simulink model "MazeGame_full"  (R2021b)
settings: Solver=FixedStepDiscrete  StartTime=0.0  StopTime=inf  FixedStep=0.001  RelTol=1e-3  EnableMultiTasking=on
PreLoadFcn:
  | initParameter;
values from neighbouring files (symbols this model uses):
  Angular2Linear = (0.054/(2*pi))    (= 0.00859436692696)    [initParameter_pendulum.m]
  cmdEl72x1_ENABLE_OPERATION = bin2dec('0000 0000 0000 1111')    [initStateMachine.m]
  cmdEl72x1_FAULT_RESET = bin2dec('0000 0000 1000 0000')    [initStateMachine.m]
  cmdEl72x1_STOP = bin2dec('0000 0000 0000 0000')    [initStateMachine.m]
  cmdEl72x1_SWITCH_ON = bin2dec('0000 0000 0000 0111')    [initStateMachine.m]
  cmdEl72x1_VOLTAGE_AND_RELEASE = bin2dec('0000 0000 0000 0110')    [initStateMachine.m]
  Counts2Voltage = (SupplyVoltage_Bottom/(32767*0.5))    (= 0.00030518509476)    [initParameter_pendulum.m]
  Counts2Voltage_top = (SupplyVoltage_Top/(32767*0.5))    (= 0.00030518509476)    [initParameter_pendulum.m]
  gearRatio_Motor1 = 1/1    (= 1)    [initParameter.m]    (also in initParameter_pendulum.m)
  increments2rad_AM8113_0F21 = 2*pi/2^20    (= 5.99211245268e-06)    [initParameter_pendulum.m]
  increments2radPerS_AM8113_0F21 = 2*pi/268435    (= 2.340672903e-05)    [initParameter_pendulum.m]
  output2Torque_AM8113_0F21 = ((1/1000)*(ratedCurrent_AM8113_0F21/sqrt(2)))*torqueConstant_AM8113_0F21    [initParameter_pendulum.m]
  PointZero_Bottom = 2476    [initParameter_pendulum.m]
  PointZero_Top = (19584 - 6*pi)    (= 19565.1504441)    [initParameter_pendulum.m]
  Safe_Distance = 0.2    [initParameter_pendulum.m]
  SupplyVoltage_Bottom = 5    [initParameter_pendulum.m]
  SupplyVoltage_Top = 5    [initParameter_pendulum.m]
  Velocity_Limit = 80*pi    (= 251.327412287)    [initParameter_pendulum.m]
  vmax_AM8113_0F21 = 90*pi    (= 282.743338823)    [initParameter_pendulum.m]
  vmin_AM8113_0F21 = -90*pi    (= -282.743338823)    [initParameter_pendulum.m]
  Voltage2Angle = SupplyVoltage_Bottom/(2*pi)    (= 0.795774715459)    [initParameter_pendulum.m]
  Voltage2Angle_top = 4.3/(2*pi)    (= 0.684366255295)    [initParameter_pendulum.m]
  Voltage2Counts = (32766/10)    (= 3276.6)    [initParameter_pendulum.m]
  x_11 = PointZero_Bottom - 1.5*pi    (= 2471.28761102)    [initParameter_pendulum.m]
  x_12 = PointZero_Bottom - (20*2*pi) + (4*2*pi)    (= 2375.46903509)    [initParameter_pendulum.m]
  x_21 = PointZero_Top + (3*2*pi)    (= 19584)    [initParameter_pendulum.m]
  x_22 = PointZero_Top + (20*2*pi)    (= 19690.8141502)    [initParameter_pendulum.m]
libraries: simulink x13, cstblocks x2
settings Model: SimulationMode=external  Creator=rauterg  LastModifiedBy=BIROMED-Lab
settings SolverCC: AlgebraicLoopSolver=TrustRegion
settings DataIOCC: LimitDataPoints=on  SaveFormat=Array  SignalLoggingSaveFormat=ModelDataLogs  ReturnWorkspaceOutputs=off
settings OptimizationCC: BlockReduction=off  ConditionallyExecuteInputs=off  UseDivisionForNetSlopeComputation=UseDivisionForReciprocalsOfIntegersOnly  OptimizeBlockIOStorage=off  BufferReuse=off  GlobalBufferReuse=off  ExpressionFolding=off  ExpressionDepthLimit=2147483647  LocalBlockOutputs=off  EfficientFloat2IntCast=on  OptimizeDataStoreBuffers=off  BusAssignmentInplaceUpdate=off
settings DebuggingCC: ConsistencyChecking=warning  SignalInfNanChecking=warning  SignalRangeChecking=error  ReadBeforeWriteMsg=EnableAllAsError  WriteAfterWriteMsg=EnableAllAsError  WriteAfterReadMsg=EnableAllAsError  AlgebraicLoopMsg=error  UnderspecifiedInitializationDetection=Classic  MergeDetectMultiDrivingBlocksExec=none  CheckExecutionContextPreStartOutputMsg=on  BlockPriorityViolationMsg=error  MinStepSizeMsg=error  TimeAdjustmentMsg=warning  SolverPrmCheckMsg=error  SigSpecEnsureSampleTimeMsg=error  CheckMatrixSingularityMsg=error  IntegerOverflowMsg=error  ParameterUnderflowMsg=error  ParameterPrecisionLossMsg=error  ParameterTunabilityLossMsg=error  UnderSpecifiedDataTypeMsg=error  UnnecessaryDatatypeConvMsg=warning  VectorMatrixConversionMsg=error  FcnCallInpInsideContextMsg=warning  SignalLabelMismatchMsg=error  UnconnectedInputMsg=error  UnconnectedOutputMsg=error  UnconnectedLineMsg=error  SFcnCompatibilityMsg=warning  UniqueDataStoreMsg=error  BusObjectLabelMismatch=error  RootOutportRequireBusObject=error  AssertControl=DisableAll  ModelReferenceIOMsg=error  ModelReferenceIOMismatchMessage=error  UnknownTsInhSupMsg=error  ModelReferenceDataLoggingMessage=error  StateNameClashWarn=warning  StrictBusMsg=ErrorOnBusTreatedAsVector  SFUnexpectedBacktrackingDiag=warning  SFNoUnconditionalDefaultTransitionDiag=warning  SFExecutionAtInitializationDiag=none  SFMachineParentedDataDiag=warning  IntegerSaturationMsg=error  ArithmeticOperatorsInVariantConditions=warning
settings HardwareCC: ProdBitPerPointer=32  ProdBitPerSizeT=32  ProdBitPerPtrDiffT=32  ProdLargestAtomicFloat=None  ProdWordSize=32  ProdLongLongMode=on  ProdHWDeviceType=Generic->32-bit x86 compatible
settings ModelReferenceCC: PropagateSignalLabelsOutOfModel=off
settings SFSimCC: SimUseLocalCustomCode=off  CustomCodeUndefinedFunction=UseInterfaceOnly  SimTargetLang=C++
settings RTWCC: Description=TwinCAT GRT Target  SystemTargetFile=TwinCatGrt.tlc  GenCodeOnly=on  TemplateMakefile=tcgrt_msbuild.tmf  GenerateReport=on  RTWUseLocalCustomCode=off  TargetLang=C++
settings CodeAppCC: ForceParamTrailComments=on  MangleLength=4  StateflowObjectComments=on  MATLABSourceComments=on
settings STFCustomTargetCC: TargetLangStandard=C++11 (ISO)  CombineOutputUpdateFcns=on  CodeInterfacePackaging=Reusable function  CPPClassGenCompliant=on  GRTInterface=off  GenerateAllocFcn=on  SystemTargetFile=TwinCatGrt.tlc
settings GRTTargetCC: TargetLangStandard=C++11 (ISO)  ParMdlRefBuildCompliant=off  CompOptLevelCompliant=off  ConcurrentExecutionCompliant=off  MatFileLogging=off  CodeInterfacePackaging=Reusable function  GenerateAllocFcn=on  UseToolchainInfoCompliant=off  ExtModeMexFile=TcExtModeClient
settings ConfigComp: CovMetricSettings=dw  CovSaveCumulativeToWorkspaceVar=on  CovSaveSingleToWorkspaceVar=on  CovExternalEMLEnable=off

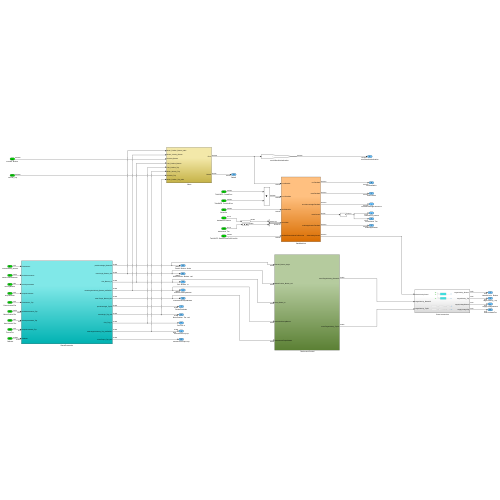
[thumbnail: Simulink's stored preview of the top-level diagram]
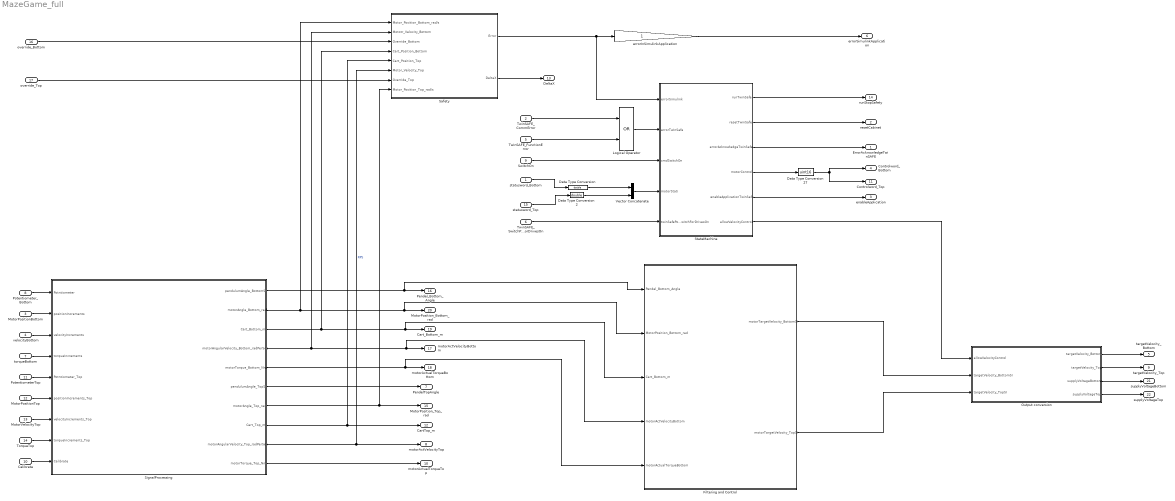
== system MazeGame_full ==
  statusword_Bottom : Inport  OutDataTypeStr=uint16
  TwinSAFE_CommError : Inport  Port=2  OutDataTypeStr=boolean
  MotorPositionBottom : Inport  Port=3  OutDataTypeStr=uint32
  velocityBottom : Inport  Port=4  OutDataTypeStr=int32
  TwinSAFE_FunctionError : Inport  Port=5  OutDataTypeStr=boolean
  TwinSAFE_SwitchPowerForDrivesOn : Inport  Port=6  OutDataTypeStr=boolean
  torqueBottom : Inport  Port=7  OutDataTypeStr=int16
  Potentiometer_Bottom : Inport  Port=8  OutDataTypeStr=int16
  SwitchOn : Inport  Port=9  OutDataTypeStr=boolean
  Calibrate : Inport  Port=10  OutDataTypeStr=boolean
  PotentiometerTop : Inport  Port=11  OutDataTypeStr=int16
  MotorPositionTop : Inport  Port=12  OutDataTypeStr=uint32
  MotorVelocityTop : Inport  Port=13  OutDataTypeStr=int32
  TorqueTop : Inport  Port=14  OutDataTypeStr=int16
  statusword_Top : Inport  Port=15  OutDataTypeStr=uint16
  override_Bottom : Inport  Port=16  OutDataTypeStr=boolean
  override_Top : Inport  Port=17  OutDataTypeStr=boolean
  Data Type Conversion : DataTypeConversion  OutDataTypeStr=double
  Data Type Conversion2 : DataTypeConversion  OutDataTypeStr=double
  Data Type Conversion27 : DataTypeConversion  OutDataTypeStr=uint16
  Filtering and Control : Subsystem
  Logical Operator : Logic  Operator=OR  AllPortsSameDT=off  OutDataTypeStr=boolean
  Output conversion : Subsystem
  Safety : Subsystem
  SignalProcessing : Subsystem
  StateMachine : Subsystem
  Vector Concatenate : Concatenate
  errorInSimulinkApplication : Gain  OutDataTypeStr=Inherit: Same as input
  ErrorAcknowledgeTwinSAFE : Outport  OutDataTypeStr=boolean  VectorParamsAs1DForOutWhenUnconnected=off
  resetCabinet : Outport  Port=2  OutDataTypeStr=boolean  VectorParamsAs1DForOutWhenUnconnected=off
  enableApplication : Outport  Port=3  OutDataTypeStr=boolean  VectorParamsAs1DForOutWhenUnconnected=off
  Controlword_Bottom : Outport  Port=4  OutDataTypeStr=uint16  VectorParamsAs1DForOutWhenUnconnected=off
  targetVelocity_Bottom : Outport  Port=5  OutDataTypeStr=int32  PortDimensions=1  VectorParamsAs1DForOutWhenUnconnected=off
  errorSimulinkApplication : Outport  Port=6  OutDataTypeStr=boolean  VectorParamsAs1DForOutWhenUnconnected=off
  PendelTopAngle : Outport  Port=7  OutDataTypeStr=double  VectorParamsAs1DForOutWhenUnconnected=off
  motorActVelocityTop : Outport  Port=8  OutDataTypeStr=double  VectorParamsAs1DForOutWhenUnconnected=off
  targetVelocity_Top : Outport  Port=9  OutDataTypeStr=int32  PortDimensions=1  VectorParamsAs1DForOutWhenUnconnected=off
  motorActualTorqueTop : Outport  Port=10  VectorParamsAs1DForOutWhenUnconnected=off
  Controlword_Top : Outport  Port=11  OutDataTypeStr=uint16  VectorParamsAs1DForOutWhenUnconnected=off
  CartTop_m : Outport  Port=12  VectorParamsAs1DForOutWhenUnconnected=off
  DeltaX : Outport  Port=13  OutDataTypeStr=double  VectorParamsAs1DForOutWhenUnconnected=off
  runStopSafety : Outport  Port=14  OutDataTypeStr=boolean  VectorParamsAs1DForOutWhenUnconnected=off
  MotorPosition_Top_rad : Outport  Port=15  OutDataTypeStr=double  VectorParamsAs1DForOutWhenUnconnected=off
  Pendel_Bottom_Angle : Outport  Port=16  OutDataTypeStr=double  VectorParamsAs1DForOutWhenUnconnected=off
  motorActVelocityBottom : Outport  Port=17  OutDataTypeStr=double  VectorParamsAs1DForOutWhenUnconnected=off
  motorActualTorqueBottom : Outport  Port=18  VectorParamsAs1DForOutWhenUnconnected=off
  Cart_Bottom_m : Outport  Port=19  VectorParamsAs1DForOutWhenUnconnected=off
  MotorPosition_Bottom_rad : Outport  Port=20  OutDataTypeStr=double  VectorParamsAs1DForOutWhenUnconnected=off
  supplyVoltageBottom : Outport  Port=21  OutDataTypeStr=int16  PortDimensions=1  VectorParamsAs1DForOutWhenUnconnected=off
  supplyVoltageTop : Outport  Port=22  OutDataTypeStr=int16  PortDimensions=1  VectorParamsAs1DForOutWhenUnconnected=off
  wires:
  TwinSAFE_CommError/1 -> Logical Operator/1
  TwinSAFE_FunctionError/1 -> Logical Operator/2
  Logical Operator/1 -> StateMachine/2(errorTwinSafe)
  SignalProcessing/4(motorAngularVelocity_Bottom_radPerSec) -> Filtering and Control/4(motorActVelocityBottom), motorActVelocityBottom/1, Safety/2(Mototr_Velocity_Bottom)
  Data Type Conversion27/1 -> Controlword_Bottom/1, Controlword_Top/1
  errorInSimulinkApplication/1 -> errorSimulinkApplication/1
  TwinSAFE_SwitchPowerForDrivesOn/1 -> StateMachine/5(twinSafePowerSwitchForDrivesOn)
  StateMachine/5(enableApplicationTwinSafe) -> enableApplication/1
  StateMachine/2(resetTwinSafe) -> resetCabinet/1
  MotorPositionBottom/1 -> SignalProcessing/2(positionIncrements)
  velocityBottom/1 -> SignalProcessing/3(velocityIncrements)
  torqueBottom/1 -> SignalProcessing/4(torqueIncrements)
  SignalProcessing/5(motorTorque_Bottom_Nm) -> Filtering and Control/5(motorActualTorqueBottom), motorActualTorqueBottom/1
  Potentiometer_Bottom/1 -> SignalProcessing/1(Potntiometer)
  SwitchOn/1 -> StateMachine/3(cmdSwitchOn)
  Calibrate/1 -> SignalProcessing/9(Calibrate)
  SignalProcessing/3(Cart_Bottom_m) -> Filtering and Control/3(Cart_Bottom_m), Cart_Bottom_m/1, Safety/4(Cart_Position_Bottom)
  SignalProcessing/1(pendulumAngle_BottomSI) -> Filtering and Control/1(Pendel_Bottom_Angle), Pendel_Bottom_Angle/1
  PotentiometerTop/1 -> SignalProcessing/5(Potntiometer_Top)
  SignalProcessing/6(pendulumAngle_TopSI) -> PendelTopAngle/1
  SignalProcessing/7(motorAngle_Top_rad) -> MotorPosition_Top_rad/1, Safety/8(Motor_Position_Top_rad/s)
  SignalProcessing/9(motorAngularVelocity_Top_radPerSec) -> motorActVelocityTop/1, Safety/6(Motor_Velocity_Top)  "RPS"
  SignalProcessing/10(motorTorque_Top_Nm) -> motorActualTorqueTop/1
  SignalProcessing/8(Cart_Top_m) -> CartTop_m/1, Safety/5(Cart_Position_Top)
  MotorPositionTop/1 -> SignalProcessing/6(positionIncrements_Top)
  MotorVelocityTop/1 -> SignalProcessing/7(velocityIncrements_Top)
  TorqueTop/1 -> SignalProcessing/8(torqueIncrements_Top)
  Data Type Conversion/1 -> Vector Concatenate/1
  statusword_Bottom/1 -> Data Type Conversion/1
  statusword_Top/1 -> Data Type Conversion2/1
  StateMachine/4(motorControl) -> Data Type Conversion27/1
  StateMachine/3(errorAcknowledgeTwinSafe) -> ErrorAcknowledgeTwinSAFE/1
  Data Type Conversion2/1 -> Vector Concatenate/2
  Safety/1(Error) -> StateMachine/1(errorSimulink), errorInSimulinkApplication/1
  Safety/2(DeltaX) -> DeltaX/1
  Vector Concatenate/1 -> StateMachine/4(motorStati)
  StateMachine/1(runTwinSafe) -> runStopSafety/1
  Output conversion/1("targetVelocity_Bottom ") -> targetVelocity_Bottom/1
  Output conversion/2(targetVelocity_Top) -> targetVelocity_Top/1
  Filtering and Control/1(motorTargetVelocity_BottomSI) -> Output conversion/2(targetVelocity_BottomSI)
  Filtering and Control/2(motorTargetVelocity_TopSI) -> Output conversion/3(targetVelocity_TopSI)
  SignalProcessing/2(motorAngle_Bottom_rad) -> MotorPosition_Bottom_rad/1, Filtering and Control/2(MotorPosition_Bottom_rad), Safety/1(Motor_Position_Bottom_rad/s)
  override_Top/1 -> Safety/7(Override_Top)
  override_Bottom/1 -> Safety/3(Override_Bottom)
  StateMachine/6(allowVelocityControl) -> Output conversion/1(allowVelocityControl)
  Output conversion/4(supplyVoltageTop) -> supplyVoltageTop/1
  Output conversion/3(supplyVoltageBottom) -> supplyVoltageBottom/1

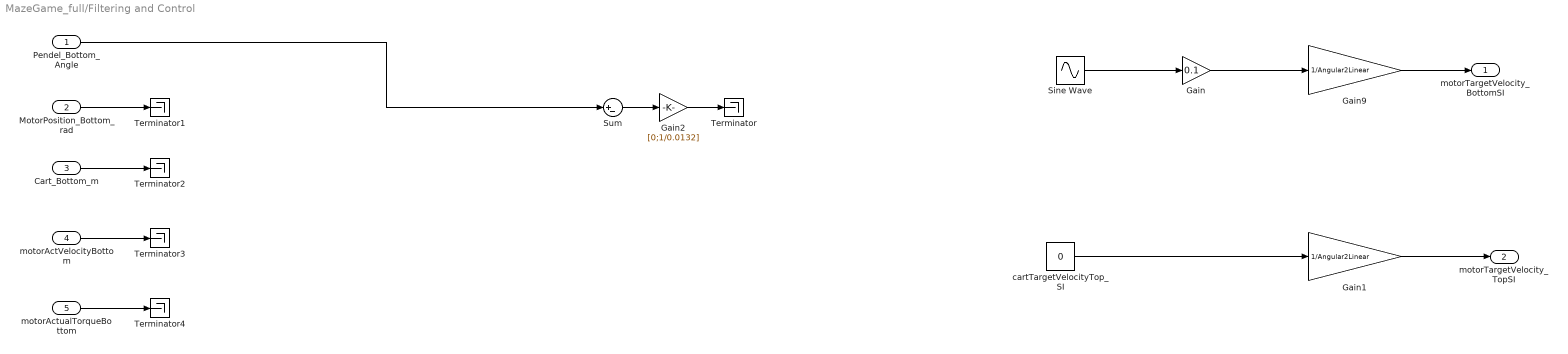
== system MazeGame_full/Filtering and Control ==
  Pendel_Bottom_Angle : Inport  OutDataTypeStr=double
  MotorPosition_Bottom_rad : Inport  Port=2  OutDataTypeStr=double
  Cart_Bottom_m : Inport  Port=3  OutDataTypeStr=double
  motorActVelocityBottom : Inport  Port=4  OutDataTypeStr=double
  motorActualTorqueBottom : Inport  Port=5  OutDataTypeStr=double
  Gain : Gain  Gain=0.1
  Gain1 : Gain  Gain=1/Angular2Linear
  Gain2 : Gain  Gain=[0;1/0.0132]
  Gain9 : Gain  Gain=1/Angular2Linear
  Sine Wave : Sin  Amplitude=0.01  Frequency=5  SampleTime=0
  Sum : Sum  Inputs=|+-
  Terminator{,1..4} (5 alike) : Terminator
  cartTargetVelocityTop_SI : Constant  Value=0
  motorTargetVelocity_BottomSI : Outport  OutDataTypeStr=double  VectorParamsAs1DForOutWhenUnconnected=off
  motorTargetVelocity_TopSI : Outport  Port=2  OutDataTypeStr=double  VectorParamsAs1DForOutWhenUnconnected=off
  wires:
  cartTargetVelocityTop_SI/1 -> Gain1/1
  Pendel_Bottom_Angle/1 -> Sum/1
  MotorPosition_Bottom_rad/1 -> Terminator1/1
  Cart_Bottom_m/1 -> Terminator2/1
  motorActVelocityBottom/1 -> Terminator3/1
  motorActualTorqueBottom/1 -> Terminator4/1
  Gain9/1 -> motorTargetVelocity_BottomSI/1
  Gain1/1 -> motorTargetVelocity_TopSI/1
  Gain/1 -> Gain9/1
  Sine Wave/1 -> Gain/1
  Sum/1 -> Gain2/1
  Gain2/1 -> Terminator/1

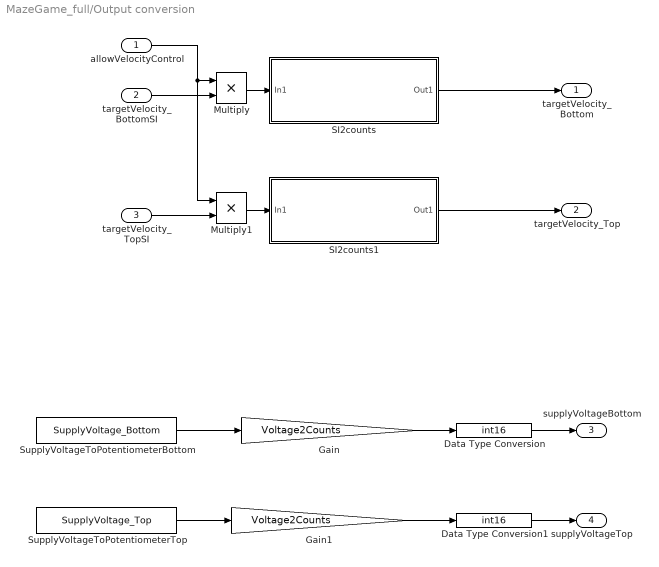
== system MazeGame_full/Output conversion ==
  allowVelocityControl : Inport
  targetVelocity_BottomSI : Inport  Port=2
  targetVelocity_TopSI : Inport  Port=3
  Data Type Conversion : DataTypeConversion  OutDataTypeStr=int16
  Data Type Conversion1 : DataTypeConversion  OutDataTypeStr=int16
  Gain : Gain  Gain=Voltage2Counts
  Gain1 : Gain  Gain=Voltage2Counts
  Multiply : Product
  Multiply1 : Product
  SI2counts : Subsystem
  SI2counts1 : Subsystem
  SupplyVoltageToPotentiometerBottom : Constant  Value=SupplyVoltage_Bottom
  SupplyVoltageToPotentiometerTop : Constant  Value=SupplyVoltage_Top
  "targetVelocity_Bottom " : Outport  OutDataTypeStr=int32  PortDimensions=1  VectorParamsAs1DForOutWhenUnconnected=off
  targetVelocity_Top : Outport  Port=2  OutDataTypeStr=int32  PortDimensions=1  VectorParamsAs1DForOutWhenUnconnected=off
  supplyVoltageBottom : Outport  Port=3  OutDataTypeStr=int16  PortDimensions=1  VectorParamsAs1DForOutWhenUnconnected=off
  supplyVoltageTop : Outport  Port=4  OutDataTypeStr=int16  PortDimensions=1  VectorParamsAs1DForOutWhenUnconnected=off
  wires:
  SI2counts1/1(Out1) -> targetVelocity_Top/1
  SI2counts/1(Out1) -> "targetVelocity_Bottom "/1
  targetVelocity_BottomSI/1 -> Multiply/2
  targetVelocity_TopSI/1 -> Multiply1/2
  Multiply/1 -> SI2counts/1(In1)
  allowVelocityControl/1 -> Multiply1/1, Multiply/1
  Multiply1/1 -> SI2counts1/1(In1)
  SupplyVoltageToPotentiometerBottom/1 -> Gain/1
  SupplyVoltageToPotentiometerTop/1 -> Gain1/1
  Gain1/1 -> Data Type Conversion1/1
  Gain/1 -> Data Type Conversion/1
  Data Type Conversion/1 -> supplyVoltageBottom/1
  Data Type Conversion1/1 -> supplyVoltageTop/1

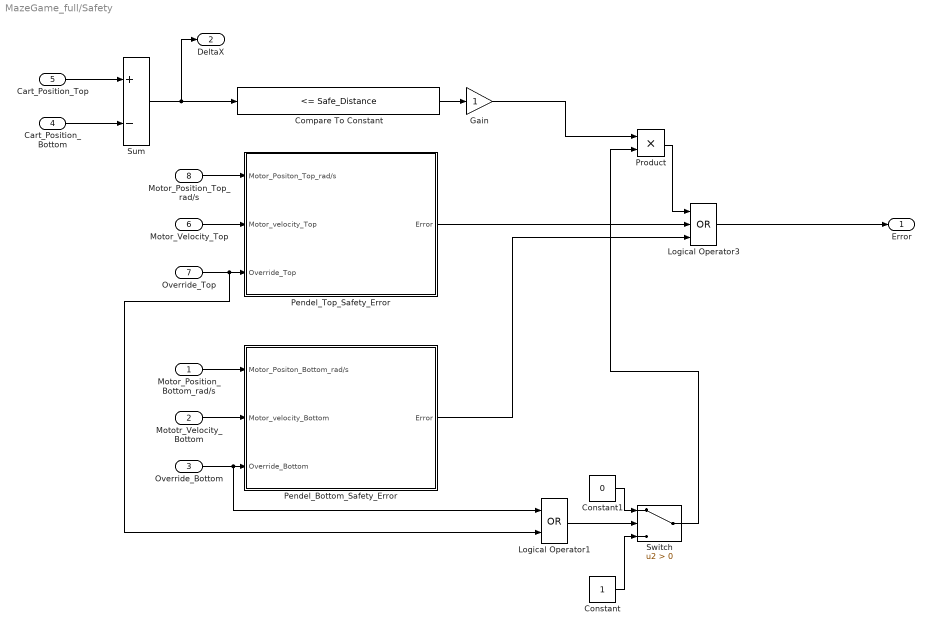
== system MazeGame_full/Safety ==
  Motor_Position_Bottom_rad/s : Inport
  Mototr_Velocity_Bottom : Inport  Port=2
  Override_Bottom : Inport  Port=3
  Cart_Position_Bottom : Inport  Port=4
  Cart_Position_Top : Inport  Port=5
  Motor_Velocity_Top : Inport  Port=6
  Override_Top : Inport  Port=7
  Motor_Position_Top_rad/s : Inport  Port=8
  Compare To Constant : simulink/Logic and Bit Operations/Compare To Constant  relop=<=  const=Safe_Distance  OutDataTypeStr=boolean
  Constant : Constant
  Constant1 : Constant  Value=0
  Gain : Gain
  Logical Operator1 : Logic  Operator=OR  AllPortsSameDT=off  OutDataTypeStr=boolean
  Logical Operator3 : Logic  Operator=OR  Inputs=3  AllPortsSameDT=off  OutDataTypeStr=boolean
  Pendel_Bottom_Safety_Error : Subsystem
  Pendel_Top_Safety_Error : Subsystem
  Product : Product
  Sum : Sum  Inputs=+-
  Switch : Switch  Criteria=u2 > Threshold
  Error : Outport  VectorParamsAs1DForOutWhenUnconnected=off
  DeltaX : Outport  Port=2  OutDataTypeStr=double  VectorParamsAs1DForOutWhenUnconnected=off
  wires:
  Logical Operator3/1 -> Error/1
  Pendel_Bottom_Safety_Error/1(Error) -> Logical Operator3/3
  Cart_Position_Top/1 -> Sum/1
  Override_Top/1 -> Logical Operator1/2, Pendel_Top_Safety_Error/3(Override_Top)
  Cart_Position_Bottom/1 -> Sum/2
  Motor_Position_Top_rad/s/1 -> Pendel_Top_Safety_Error/1(Motor_Positon_Top_rad/s)
  Override_Bottom/1 -> Logical Operator1/1, Pendel_Bottom_Safety_Error/3(Override_Bottom)
  Motor_Position_Bottom_rad/s/1 -> Pendel_Bottom_Safety_Error/1(Motor_Positon_Bottom_rad/s)
  Motor_Velocity_Top/1 -> Pendel_Top_Safety_Error/2(Motor_velocity_Top)
  Mototr_Velocity_Bottom/1 -> Pendel_Bottom_Safety_Error/2(Motor_velocity_Bottom)
  Compare To Constant/1 -> Gain/1
  Sum/1 -> DeltaX/1, Compare To Constant/1
  Pendel_Top_Safety_Error/1(Error) -> Logical Operator3/2
  Logical Operator1/1 -> Switch/2
  Product/1 -> Logical Operator3/1
  Constant/1 -> Switch/3
  Constant1/1 -> Switch/1
  Switch/1 -> Product/2
  Gain/1 -> Product/1

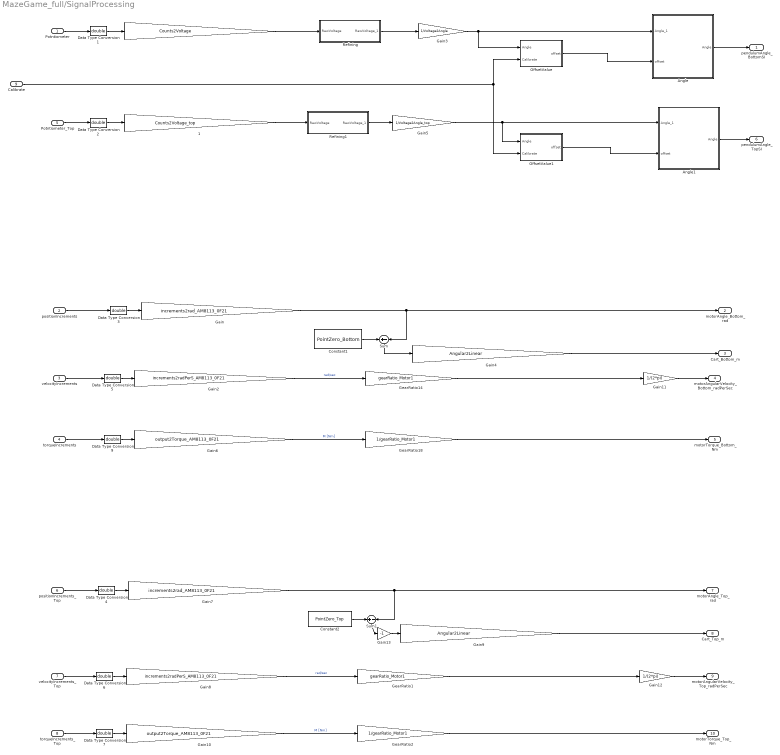
== system MazeGame_full/SignalProcessing ==
  Potntiometer : Inport
  positionIncrements : Inport  Port=2
  velocityIncrements : Inport  Port=3
  torqueIncrements : Inport  Port=4
  Potntiometer_Top : Inport  Port=5
  positionIncrements_Top : Inport  Port=6  OutDataTypeStr=uint32
  velocityIncrements_Top : Inport  Port=7  OutDataTypeStr=int32
  torqueIncrements_Top : Inport  Port=8  OutDataTypeStr=int16
  Calibrate : Inport  Port=9  OutDataTypeStr=boolean
  " " : Gain  Gain=Counts2Voltage
  " 1" : Gain  Gain=Counts2Voltage_top
  Angle : Subsystem
  Angle1 : Subsystem
  Constant1 : Constant  Value=PointZero_Bottom
  Constant2 : Constant  Value=PointZero_Top
  Data Type Conversion{1..7,9} (8 alike) : DataTypeConversion  OutDataTypeStr=double
  Gain : Gain  Gain=increments2rad_AM8113_0F21
  Gain10 : Gain  Gain=output2Torque_AM8113_0F21
  Gain11 : Gain  Gain=1/(2*pi)
  Gain12 : Gain  Gain=1/(2*pi)
  Gain13 : Gain  Gain=-1
  Gain2 : Gain  Gain=increments2radPerS_AM8113_0F21
  Gain3 : Gain  Gain=1/Voltage2Angle
  Gain4 : Gain  Gain=Angular2Linear
  Gain5 : Gain  Gain=1/Voltage2Angle_top
  Gain6 : Gain  Gain=output2Torque_AM8113_0F21
  Gain7 : Gain  Gain=increments2rad_AM8113_0F21
  Gain8 : Gain  Gain=increments2radPerS_AM8113_0F21
  Gain9 : Gain  Gain=Angular2Linear
  GearRatio1 : Gain  Gain=gearRatio_Motor1
  GearRatio14 : Gain  Gain=gearRatio_Motor1
  GearRatio18 : Gain  Gain=1/gearRatio_Motor1
  GearRatio2 : Gain  Gain=1/gearRatio_Motor1
  OffsetValue : Subsystem
  OffsetValue1 : Subsystem
  Refining : Subsystem
  Refining1 : Subsystem
  Sum : Sum  Inputs=+-
  Sum1 : Sum  Inputs=+-
  pendulumAngle_BottomSI : Outport  VectorParamsAs1DForOutWhenUnconnected=off
  motorAngle_Bottom_rad : Outport  Port=2  VectorParamsAs1DForOutWhenUnconnected=off
  Cart_Bottom_m : Outport  Port=3  VectorParamsAs1DForOutWhenUnconnected=off
  motorAngularVelocity_Bottom_radPerSec : Outport  Port=4  VectorParamsAs1DForOutWhenUnconnected=off
  motorTorque_Bottom_Nm : Outport  Port=5  VectorParamsAs1DForOutWhenUnconnected=off
  pendulumAngle_TopSI : Outport  Port=6  VectorParamsAs1DForOutWhenUnconnected=off
  motorAngle_Top_rad : Outport  Port=7  VectorParamsAs1DForOutWhenUnconnected=off
  Cart_Top_m : Outport  Port=8  VectorParamsAs1DForOutWhenUnconnected=off
  motorAngularVelocity_Top_radPerSec : Outport  Port=9  VectorParamsAs1DForOutWhenUnconnected=off
  motorTorque_Top_Nm : Outport  Port=10  VectorParamsAs1DForOutWhenUnconnected=off
  wires:
  velocityIncrements/1 -> Data Type Conversion5/1
  Gain2/1 -> GearRatio14/1  "rad/sec"
  GearRatio14/1 -> Gain11/1
  Data Type Conversion9/1 -> Gain6/1
  Data Type Conversion5/1 -> Gain2/1
  torqueIncrements/1 -> Data Type Conversion9/1
  Gain6/1 -> GearRatio18/1  "M [Nm]"
  GearRatio18/1 -> motorTorque_Bottom_Nm/1
  Potntiometer/1 -> Data Type Conversion1/1
  Data Type Conversion1/1 -> " "/1
  Calibrate/1 -> OffsetValue/2(Calibrate), OffsetValue1/2(Calibrate)
  OffsetValue/1(offset) -> Angle/2(offset)
  Angle/1(Angle) -> pendulumAngle_BottomSI/1
  Gain3/1 -> OffsetValue/1(Angle), Angle/1(Angle_1)
  " "/1 -> Refining/1(RawVoltage)
  Refining/1(RawVoltage_1) -> Gain3/1
  Angle1/1(Angle) -> pendulumAngle_TopSI/1
  Potntiometer_Top/1 -> Data Type Conversion2/1
  Refining1/1(RawVoltage_1) -> Gain5/1
  Data Type Conversion2/1 -> " 1"/1
  " 1"/1 -> Refining1/1(RawVoltage)
  Gain5/1 -> Angle1/1(Angle_1), OffsetValue1/1(Angle)
  OffsetValue1/1(offset) -> Angle1/2(offset)
  Gain7/1 -> Sum1/2, motorAngle_Top_rad/1
  Sum1/1 -> Gain13/1
  GearRatio2/1 -> motorTorque_Top_Nm/1
  Constant2/1 -> Sum1/1
  positionIncrements_Top/1 -> Data Type Conversion4/1
  Gain9/1 -> Cart_Top_m/1
  torqueIncrements_Top/1 -> Data Type Conversion7/1
  Data Type Conversion7/1 -> Gain10/1
  Data Type Conversion4/1 -> Gain7/1
  Gain8/1 -> GearRatio1/1  "rad/sec"
  Gain10/1 -> GearRatio2/1  "M [Nm]"
  Data Type Conversion6/1 -> Gain8/1
  GearRatio1/1 -> Gain12/1
  velocityIncrements_Top/1 -> Data Type Conversion6/1
  Gain11/1 -> motorAngularVelocity_Bottom_radPerSec/1
  Gain12/1 -> motorAngularVelocity_Top_radPerSec/1
  Gain13/1 -> Gain9/1
  Gain4/1 -> Cart_Bottom_m/1
  Sum/1 -> Gain4/1
  Constant1/1 -> Sum/1
  positionIncrements/1 -> Data Type Conversion3/1
  Gain/1 -> Sum/2, motorAngle_Bottom_rad/1
  Data Type Conversion3/1 -> Gain/1

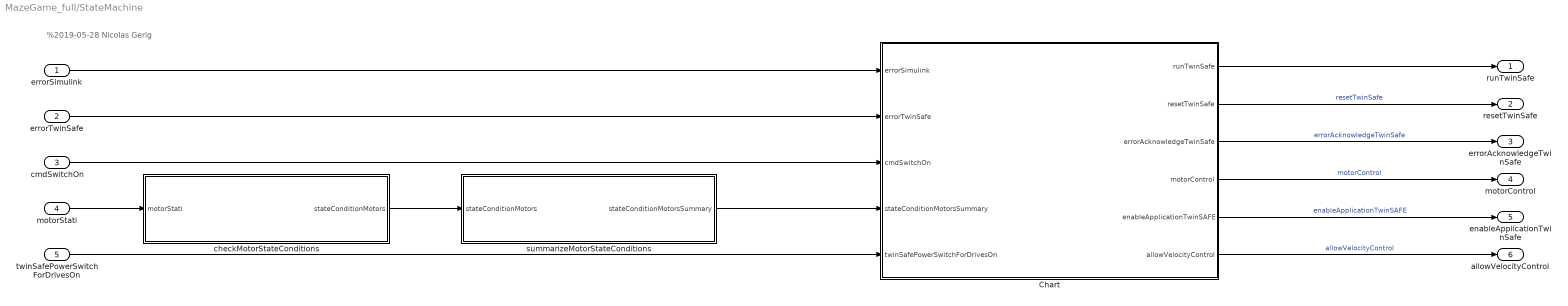
== system MazeGame_full/StateMachine ==
  note: %2019-05-28 Nicolas Gerig
  errorSimulink : Inport  OutDataTypeStr=boolean  PortDimensions=1  SampleTime=0
  errorTwinSafe : Inport  Port=2  OutDataTypeStr=boolean  PortDimensions=1  SampleTime=0
  cmdSwitchOn : Inport  Port=3  OutDataTypeStr=boolean  PortDimensions=1
  motorStati : Inport  Port=4  OutDataTypeStr=double  SampleTime=0
  twinSafePowerSwitchForDrivesOn : Inport  Port=5  OutDataTypeStr=boolean  PortDimensions=1  SampleTime=0
  Chart : Stateflow chart  TreatAsAtomicUnit=on
  checkMotorStateConditions : MATLAB Function  TreatAsAtomicUnit=on
  summarizeMotorStateConditions : MATLAB Function  TreatAsAtomicUnit=on
  runTwinSafe : Outport  OutDataTypeStr=boolean  PortDimensions=1  SampleTime=0  VectorParamsAs1DForOutWhenUnconnected=off
  resetTwinSafe : Outport  Port=2  OutDataTypeStr=boolean  PortDimensions=1  SampleTime=0  VectorParamsAs1DForOutWhenUnconnected=off
  errorAcknowledgeTwinSafe : Outport  Port=3  OutDataTypeStr=boolean  PortDimensions=1  SampleTime=0  VectorParamsAs1DForOutWhenUnconnected=off
  motorControl : Outport  Port=4  OutDataTypeStr=double  PortDimensions=1  SampleTime=0  VectorParamsAs1DForOutWhenUnconnected=off
  enableApplicationTwinSafe : Outport  Port=5  OutDataTypeStr=boolean  PortDimensions=1  SampleTime=0  VectorParamsAs1DForOutWhenUnconnected=off
  allowVelocityControl : Outport  Port=6  OutDataTypeStr=boolean  PortDimensions=1  SampleTime=0  VectorParamsAs1DForOutWhenUnconnected=off
  wires:
  checkMotorStateConditions/1(stateConditionMotors) -> summarizeMotorStateConditions/1(stateConditionMotors)
  summarizeMotorStateConditions/1(stateConditionMotorsSummary) -> Chart/4(stateConditionMotorsSummary)
  Chart/2(resetTwinSafe) -> resetTwinSafe/1  "resetTwinSafe"
  twinSafePowerSwitchForDrivesOn/1 -> Chart/5(twinSafePowerSwitchForDrivesOn)
  Chart/4(motorControl) -> motorControl/1  "motorControl"
  Chart/3(errorAcknowledgeTwinSafe) -> errorAcknowledgeTwinSafe/1  "errorAcknowledgeTwinSafe"
  cmdSwitchOn/1 -> Chart/3(cmdSwitchOn)
  Chart/6(allowVelocityControl) -> allowVelocityControl/1  "allowVelocityControl"
  errorTwinSafe/1 -> Chart/2(errorTwinSafe)
  Chart/5(enableApplicationTwinSAFE) -> enableApplicationTwinSafe/1  "enableApplicationTwinSAFE"
  errorSimulink/1 -> Chart/1(errorSimulink)
  motorStati/1 -> checkMotorStateConditions/1(motorStati)
  Chart/1(runTwinSafe) -> runTwinSafe/1

== system MazeGame_full/Output conversion/SI2counts ==
  In1 : Inport
  Data Type Conversion7 : DataTypeConversion  OutDataTypeStr=int32
  Gain4 : Gain  Gain=1/increments2radPerS_AM8113_0F21
  GearRatio : Gain  Gain=1/gearRatio_Motor1
  Saturation1 : Saturate  UpperLimit=vmax_AM8113_0F21  LowerLimit=vmin_AM8113_0F21
  Out1 : Outport  VectorParamsAs1DForOutWhenUnconnected=off
  wires:
  Gain4/1 -> Data Type Conversion7/1
  GearRatio/1 -> Saturation1/1
  Data Type Conversion7/1 -> Out1/1
  Saturation1/1 -> Gain4/1
  In1/1 -> GearRatio/1

== system MazeGame_full/Output conversion/SI2counts1 ==
  In1 : Inport
  Data Type Conversion7 : DataTypeConversion  OutDataTypeStr=int32
  Gain4 : Gain  Gain=1/increments2radPerS_AM8113_0F21
  GearRatio : Gain  Gain=1/gearRatio_Motor1
  Saturation1 : Saturate  UpperLimit=vmax_AM8113_0F21  LowerLimit=vmin_AM8113_0F21
  Out1 : Outport  VectorParamsAs1DForOutWhenUnconnected=off
  wires:
  Gain4/1 -> Data Type Conversion7/1
  GearRatio/1 -> Saturation1/1
  Data Type Conversion7/1 -> Out1/1
  Saturation1/1 -> Gain4/1
  In1/1 -> GearRatio/1

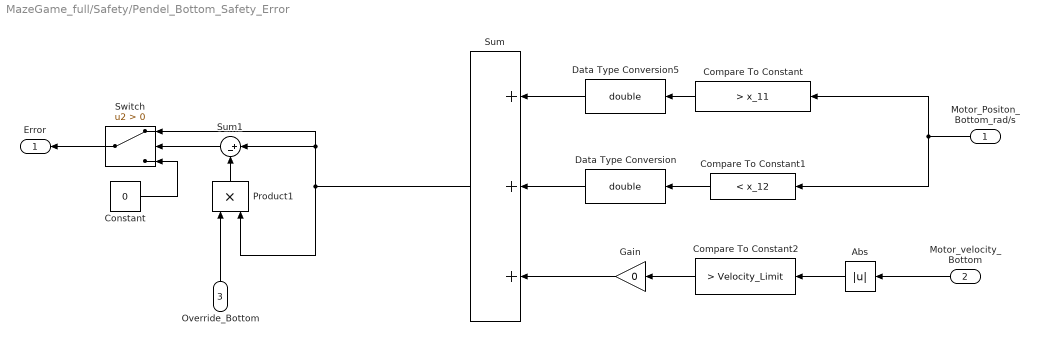
== system MazeGame_full/Safety/Pendel_Bottom_Safety_Error ==
  Motor_Positon_Bottom_rad/s : Inport
  Motor_velocity_Bottom : Inport  Port=2
  Override_Bottom : Inport  Port=3
  Abs : Abs
  Compare To Constant : simulink/Logic and Bit Operations/Compare To Constant  relop=>  const=x_11  OutDataTypeStr=boolean
  Compare To Constant1 : simulink/Logic and Bit Operations/Compare To Constant  relop=<  const=x_12  OutDataTypeStr=boolean
  Compare To Constant2 : simulink/Logic and Bit Operations/Compare To Constant  relop=>  const=Velocity_Limit  OutDataTypeStr=boolean
  Constant : Constant  Value=0
  Data Type Conversion : DataTypeConversion  OutDataTypeStr=double
  Data Type Conversion5 : DataTypeConversion  OutDataTypeStr=double
  Gain : Gain  Gain=0
  Product1 : Product
  Sum : Sum  Inputs=+++
  Sum1 : Sum  Inputs=|+-
  Switch : Switch  Criteria=u2 > Threshold
  Error : Outport  VectorParamsAs1DForOutWhenUnconnected=off
  wires:
  Abs/1 -> Compare To Constant2/1
  Compare To Constant1/1 -> Data Type Conversion/1
  Compare To Constant/1 -> Data Type Conversion5/1
  Data Type Conversion5/1 -> Sum/1
  Data Type Conversion/1 -> Sum/2
  Compare To Constant2/1 -> Gain/1
  Sum1/1 -> Switch/2
  Sum/1 -> Product1/2, Sum1/1, Switch/1
  Gain/1 -> Sum/3
  Constant/1 -> Switch/3
  Product1/1 -> Sum1/2
  Switch/1 -> Error/1
  Override_Bottom/1 -> Product1/1
  Motor_velocity_Bottom/1 -> Abs/1
  Motor_Positon_Bottom_rad/s/1 -> Compare To Constant/1, Compare To Constant1/1

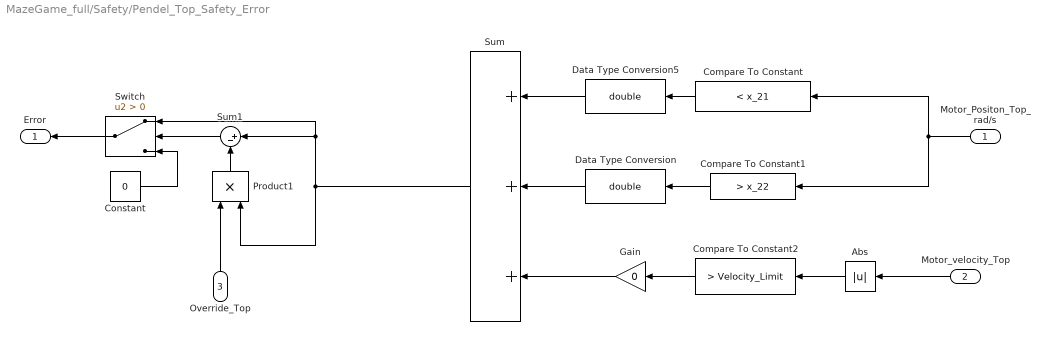
== system MazeGame_full/Safety/Pendel_Top_Safety_Error ==
  Motor_Positon_Top_rad/s : Inport
  Motor_velocity_Top : Inport  Port=2
  Override_Top : Inport  Port=3
  Abs : Abs
  Compare To Constant : simulink/Logic and Bit Operations/Compare To Constant  relop=<  const=x_21  OutDataTypeStr=boolean
  Compare To Constant1 : simulink/Logic and Bit Operations/Compare To Constant  relop=>  const=x_22  OutDataTypeStr=boolean
  Compare To Constant2 : simulink/Logic and Bit Operations/Compare To Constant  relop=>  const=Velocity_Limit  OutDataTypeStr=boolean
  Constant : Constant  Value=0
  Data Type Conversion : DataTypeConversion  OutDataTypeStr=double
  Data Type Conversion5 : DataTypeConversion  OutDataTypeStr=double
  Gain : Gain  Gain=0
  Product1 : Product
  Sum : Sum  Inputs=+++
  Sum1 : Sum  Inputs=|+-
  Switch : Switch  Criteria=u2 > Threshold
  Error : Outport  VectorParamsAs1DForOutWhenUnconnected=off
  wires:
  Abs/1 -> Compare To Constant2/1
  Compare To Constant1/1 -> Data Type Conversion/1
  Compare To Constant/1 -> Data Type Conversion5/1
  Data Type Conversion5/1 -> Sum/1
  Data Type Conversion/1 -> Sum/2
  Compare To Constant2/1 -> Gain/1
  Sum1/1 -> Switch/2
  Sum/1 -> Product1/2, Sum1/1, Switch/1
  Gain/1 -> Sum/3
  Constant/1 -> Switch/3
  Product1/1 -> Sum1/2
  Switch/1 -> Error/1
  Override_Top/1 -> Product1/1
  Motor_velocity_Top/1 -> Abs/1
  Motor_Positon_Top_rad/s/1 -> Compare To Constant/1, Compare To Constant1/1

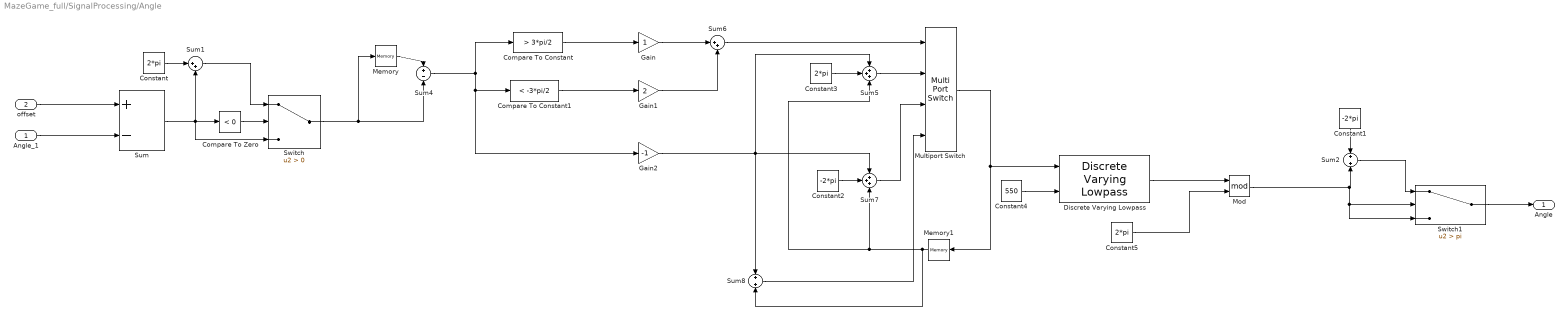
== system MazeGame_full/SignalProcessing/Angle ==
  Angle_1 : Inport
  offset : Inport  Port=2
  Compare To Constant : simulink/Logic and Bit Operations/Compare To Constant  relop=>  const=3*pi/2  OutDataTypeStr=boolean
  Compare To Constant1 : simulink/Logic and Bit Operations/Compare To Constant  relop=<  const=-3*pi/2  OutDataTypeStr=boolean
  Compare To Zero : simulink/Logic and Bit Operations/Compare To Zero  relop=<  OutDataTypeStr=boolean
  Constant : Constant  Value=2*pi
  Constant1 : Constant  Value=-2*pi
  Constant2 : Constant  Value=-2*pi
  Constant3 : Constant  Value=2*pi
  Constant4 : Constant  Value=550
  Constant5 : Constant  Value=2*pi
  Discrete Varying Lowpass : cstblocks/Linear Parameter Varying/Discrete Varying Lowpass  N=1  w0=0  Ts=0.001
      settings: SourceProductBaseCode=CT
  Gain : Gain
  Gain1 : Gain  Gain=2
  Gain2 : Gain  Gain=-1
  Memory : Memory
  Memory1 : Memory
  Mod : Math  Operator=mod  SignedPower=on  SaturateOnIntegerOverflow=on
  Multiport Switch : MultiPortSwitch
  Sum : Sum  Inputs=+-
  Sum1 : Sum  Inputs=|++
  Sum2 : Sum
  Sum4 : Sum  Inputs=+-
  Sum5 : Sum  Inputs=+++
  Sum6 : Sum  Inputs=|++
  Sum7 : Sum  Inputs=+++
  Sum8 : Sum
  Switch : Switch  Criteria=u2 > Threshold
  Switch1 : Switch  Criteria=u2 > Threshold  Threshold=pi
  Angle : Outport  VectorParamsAs1DForOutWhenUnconnected=off
  wires:
  Sum/1 -> Compare To Zero/1, Switch/3, Sum1/2
  offset/1 -> Sum/1
  Compare To Zero/1 -> Switch/2
  Constant/1 -> Sum1/1
  Sum1/1 -> Switch/1
  Switch/1 -> Memory/1, Sum4/2
  Constant1/1 -> Sum2/1
  Sum2/1 -> Switch1/1
  Angle_1/1 -> Sum/2
  Memory/1 -> Sum4/1
  Sum4/1 -> Gain2/1, Compare To Constant1/1, Compare To Constant/1
  Constant3/1 -> Sum5/2
  Compare To Constant/1 -> Gain/1
  Compare To Constant1/1 -> Gain1/1
  Gain/1 -> Sum6/1
  Gain1/1 -> Sum6/2
  Sum6/1 -> Multiport Switch/1
  Sum5/1 -> Multiport Switch/2
  Gain2/1 -> Sum7/1, Sum5/1, Sum8/1
  Constant2/1 -> Sum7/2
  Memory1/1 -> Sum5/3, Sum7/3, Sum8/2
  Sum7/1 -> Multiport Switch/3
  Sum8/1 -> Multiport Switch/4
  Multiport Switch/1 -> Memory1/1, Discrete Varying Lowpass/1
  Discrete Varying Lowpass/1 -> Mod/1
  Constant4/1 -> Discrete Varying Lowpass/2
  Constant5/1 -> Mod/2
  Mod/1 -> Switch1/3, Switch1/2, Sum2/2
  Switch1/1 -> Angle/1

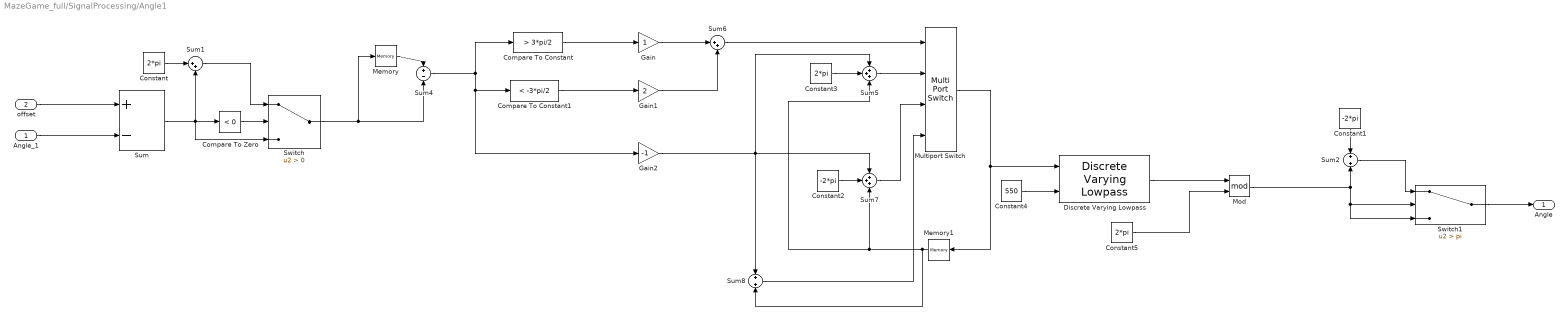
== system MazeGame_full/SignalProcessing/Angle1 ==
  Angle_1 : Inport
  offset : Inport  Port=2
  Compare To Constant : simulink/Logic and Bit Operations/Compare To Constant  relop=>  const=3*pi/2  OutDataTypeStr=boolean
  Compare To Constant1 : simulink/Logic and Bit Operations/Compare To Constant  relop=<  const=-3*pi/2  OutDataTypeStr=boolean
  Compare To Zero : simulink/Logic and Bit Operations/Compare To Zero  relop=<  OutDataTypeStr=boolean
  Constant : Constant  Value=2*pi
  Constant1 : Constant  Value=-2*pi
  Constant2 : Constant  Value=-2*pi
  Constant3 : Constant  Value=2*pi
  Constant4 : Constant  Value=550
  Constant5 : Constant  Value=2*pi
  Discrete Varying Lowpass : cstblocks/Linear Parameter Varying/Discrete Varying Lowpass  N=1  w0=0  Ts=0.001
      settings: SourceProductBaseCode=CT
  Gain : Gain
  Gain1 : Gain  Gain=2
  Gain2 : Gain  Gain=-1
  Memory : Memory
  Memory1 : Memory
  Mod : Math  Operator=mod  SignedPower=on  SaturateOnIntegerOverflow=on
  Multiport Switch : MultiPortSwitch
  Sum : Sum  Inputs=+-
  Sum1 : Sum  Inputs=|++
  Sum2 : Sum
  Sum4 : Sum  Inputs=+-
  Sum5 : Sum  Inputs=+++
  Sum6 : Sum  Inputs=|++
  Sum7 : Sum  Inputs=+++
  Sum8 : Sum
  Switch : Switch  Criteria=u2 > Threshold
  Switch1 : Switch  Criteria=u2 > Threshold  Threshold=pi
  Angle : Outport  VectorParamsAs1DForOutWhenUnconnected=off
  wires:
  Sum/1 -> Compare To Zero/1, Switch/3, Sum1/2
  offset/1 -> Sum/1
  Compare To Zero/1 -> Switch/2
  Constant/1 -> Sum1/1
  Sum1/1 -> Switch/1
  Switch1/1 -> Angle/1
  Switch/1 -> Memory/1, Sum4/2
  Constant1/1 -> Sum2/1
  Sum2/1 -> Switch1/1
  Angle_1/1 -> Sum/2
  Memory/1 -> Sum4/1
  Sum4/1 -> Gain2/1, Compare To Constant1/1, Compare To Constant/1
  Constant3/1 -> Sum5/2
  Compare To Constant/1 -> Gain/1
  Compare To Constant1/1 -> Gain1/1
  Gain/1 -> Sum6/1
  Gain1/1 -> Sum6/2
  Sum6/1 -> Multiport Switch/1
  Sum5/1 -> Multiport Switch/2
  Gain2/1 -> Sum7/1, Sum5/1, Sum8/1
  Constant2/1 -> Sum7/2
  Memory1/1 -> Sum5/3, Sum7/3, Sum8/2
  Sum7/1 -> Multiport Switch/3
  Sum8/1 -> Multiport Switch/4
  Multiport Switch/1 -> Memory1/1, Discrete Varying Lowpass/1
  Discrete Varying Lowpass/1 -> Mod/1
  Constant4/1 -> Discrete Varying Lowpass/2
  Constant5/1 -> Mod/2
  Mod/1 -> Sum2/2, Switch1/3, Switch1/2

== system MazeGame_full/SignalProcessing/OffsetValue ==
  Angle : Inport
  Calibrate : Inport  Port=2  OutDataTypeStr=boolean
  Data Type Conversion2 : DataTypeConversion  OutDataTypeStr=boolean
  Data Type Conversion7 : DataTypeConversion  OutDataTypeStr=double
  MATLAB Function : MATLAB Function  TreatAsAtomicUnit=on
  Terminator : Terminator
  offset : Outport  VectorParamsAs1DForOutWhenUnconnected=off
  wires:
  Data Type Conversion7/1 -> MATLAB Function/2(i)
  Calibrate/1 -> Data Type Conversion7/1
  MATLAB Function/2(ready) -> Data Type Conversion2/1
  Data Type Conversion2/1 -> Terminator/1
  Angle/1 -> MATLAB Function/1(u)
  MATLAB Function/1(y) -> offset/1

== system MazeGame_full/SignalProcessing/OffsetValue1 ==
  Angle : Inport
  Calibrate : Inport  Port=2  OutDataTypeStr=boolean
  Data Type Conversion2 : DataTypeConversion  OutDataTypeStr=boolean
  Data Type Conversion7 : DataTypeConversion  OutDataTypeStr=double
  MATLAB_Top : MATLAB Function  TreatAsAtomicUnit=on
  Terminator : Terminator
  offset : Outport  VectorParamsAs1DForOutWhenUnconnected=off
  wires:
  Data Type Conversion7/1 -> MATLAB_Top/2(i)
  Calibrate/1 -> Data Type Conversion7/1
  MATLAB_Top/2(ready) -> Data Type Conversion2/1
  Data Type Conversion2/1 -> Terminator/1
  Angle/1 -> MATLAB_Top/1(u)
  MATLAB_Top/1(y) -> offset/1

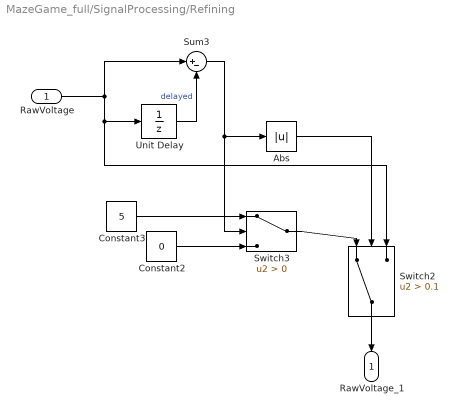
== system MazeGame_full/SignalProcessing/Refining ==
  RawVoltage : Inport
  Abs : Abs
  Constant2 : Constant  Value=0
  Constant3 : Constant  Value=5
  Sum3 : Sum  Inputs=|+-
  Switch2 : Switch  Criteria=u2 > Threshold  Threshold=0.1
  Switch3 : Switch  Criteria=u2 > Threshold
  Unit Delay : UnitDelay  SampleTime=-1  HasFrameUpgradeWarning=on
  RawVoltage_1 : Outport  VectorParamsAs1DForOutWhenUnconnected=off
  wires:
  Unit Delay/1 -> Sum3/2  "delayed"
  Abs/1 -> Switch2/2
  Switch3/1 -> Switch2/1
  Sum3/1 -> Abs/1, Switch3/2
  Constant2/1 -> Switch3/3
  Constant3/1 -> Switch3/1
  Switch2/1 -> RawVoltage_1/1
  RawVoltage/1 -> Sum3/1, Switch2/3, Unit Delay/1

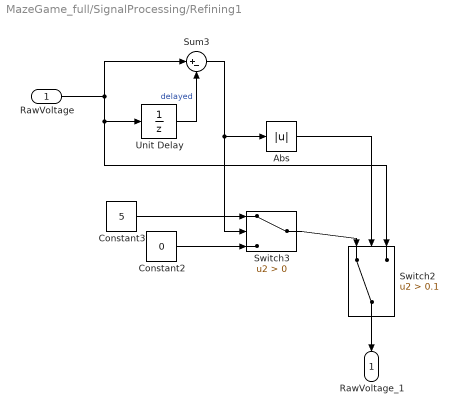
== system MazeGame_full/SignalProcessing/Refining1 ==
  RawVoltage : Inport
  Abs : Abs
  Constant2 : Constant  Value=0
  Constant3 : Constant  Value=5
  Sum3 : Sum  Inputs=|+-
  Switch2 : Switch  Criteria=u2 > Threshold  Threshold=0.1
  Switch3 : Switch  Criteria=u2 > Threshold
  Unit Delay : UnitDelay  SampleTime=-1  HasFrameUpgradeWarning=on
  RawVoltage_1 : Outport  VectorParamsAs1DForOutWhenUnconnected=off
  wires:
  Unit Delay/1 -> Sum3/2  "delayed"
  Abs/1 -> Switch2/2
  Switch3/1 -> Switch2/1
  Sum3/1 -> Abs/1, Switch3/2
  Constant2/1 -> Switch3/3
  Constant3/1 -> Switch3/1
  Switch2/1 -> RawVoltage_1/1
  RawVoltage/1 -> Sum3/1, Switch2/3, Unit Delay/1

== matlab function MazeGame_full/SignalProcessing/OffsetValue/MATLAB Function ==
  data: u input; y output; i input; ready output
function [y,ready] = fcn(u,i)
persistent angle ready1 ;
if isempty (angle)
    angle = 0;
    ready1 = 0;
    
    
end
if i == 1
    
    
        
        
    angle  = u;
    ready1 = 1;    
    
    
end
y = angle; ready = ready1;

== matlab function MazeGame_full/SignalProcessing/OffsetValue1/MATLAB_Top ==
  data: u input; y output; i input; ready output
function [y,ready] = fcn(u,i)
persistent angle ready1 ;
if isempty (angle)
    angle = 0;
    ready1 = 0;
    
    
end
if i == 1
    
    
        
        
    angle  = u;
    ready1 = 1;    
    
    
end
y = angle; ready = ready1;

== matlab function MazeGame_full/StateMachine/checkMotorStateConditions ==
  data: motorStati input; stateConditionMotors output Bus: StateConditionMotors size=1
function stateConditionMotors = checkMotorStateConditions(motorStati)
%2019-05-28 Nicolas Gerig

%% outputs:
stateConditionMotors.bSwitchOnDisabled = checkMotorsSwitchOnDisabled(motorStati);
stateConditionMotors.bReadyToSwitchOn = checkMotorsReadyToSwitchOn(motorStati);
stateConditionMotors.bSwitchedOn = checkMotorsSwitchedOn(motorStati);
stateConditionMotors.bOperationEnabled = checkMotorsOperationEnabled(motorStati);

%% checking Status words for state
    function bResults = checkMotorsSwitchOnDisabled(motorStati)
        
        bResults = false( length(motorStati), 1 );
        
        for i=1:length(motorStati)
            bResults(i) = checkEl72x1_SWITCH_ON_DISABLED( motorStati(i) );
        end
        
    end

    function bResults = checkMotorsReadyToSwitchOn(motorStati)
        
        bResults = false( length(motorStati), 1 );
        
        for i=1:length(motorStati)
            bResults(i) = checkEl72x1_READY_TO_SWITCH_ON( motorStati(i) );
        end        
    end
		
	function bResults = checkMotorsSwitchedOn(motorStati)
        
        bResults = false( length(motorStati), 1 );
        
        for i=1:length(motorStati)
            bResults(i) = checkEl72x1_SWITCHED_ON( motorStati(i) );
        end        
    end
	
	function bResults = checkMotorsOperationEnabled(motorStati)
        
        bResults = false( length(motorStati), 1 );
        
        for i=1:length(motorStati)
            bResults(i) = checkEl72x1_OPERATION_ENABLED( motorStati(i) );
        end
    end
	
%% Status word checks EL72X1:
%"6010:01 Statusword" https://download.beckhoff.com/download/document/io/ethercat-terminals/el72x1-001xde.pdf

    function bResult = checkEl72x1_SWITCH_ON_DISABLED(motorStatus)
        bResult = checkIfBit_TRUE( motorStatus, 6);% EL72X1: bit6 switch on disabled
    end
		
    function bResult = checkEl72x1_READY_TO_SWITCH_ON(motorStatus)
        bResult = ( checkIfBit_TRUE( motorStatus, 0 ) ...% ready to switch on (bit0)
            && checkIfBit_FALSE( motorStatus, 1 ) ...% not switched on (bit1)
            && checkIfBit_FALSE( motorStatus, 2 ) ...% not operation enabled (bit2)
            && checkIfBit_FALSE( motorStatus, 3 ) ...% not fault (bit3)
            && checkIfBit_TRUE( motorStatus, 5 ) ...% quick stop (inverse bit5) (:= true means released)
            && checkIfBit_FALSE( motorStatus, 6 ) );% not switch on disabled (bit6)
    end
	
	function bResult = checkEl72x1_SWITCHED_ON(motorStatus)
        bResult = ( checkIfBit_TRUE( motorStatus, 0 ) ...% ready to switch on (bit0)
            && checkIfBit_TRUE( motorStatus, 1 ) ...% switched on (bit1)
            && checkIfBit_FALSE( motorStatus, 2 ) ...% not operation enabled (bit2)
            && checkIfBit_FALSE( motorStatus, 3 ) ...% not fault (bit3)
            && checkIfBit_TRUE( motorStatus, 5 ) ...% quick stop (inverse bit5) (:= true means released)
            && checkIfBit_FALSE( motorStatus, 6 ) );% not switch on disabled (bit6)
    end

	function bResult = checkEl72x1_OPERATION_ENABLED(motorStatus)
        bResult = ( checkIfBit_TRUE( motorStatus, 0 ) ...% ready to switch on (bit0)
            && checkIfBit_TRUE( motorStatus, 1 ) ...% switched on (bit1)
            && checkIfBit_TRUE( motorStatus, 2 ) ...% operation enabled (bit2)
            && checkIfBit_FALSE( motorStatus, 3 ) ...% not fault (bit3)
            && checkIfBit_TRUE( motorStatus, 5 ) ...% quick stop (inverse bit5) (:= true means released)
            && checkIfBit_FALSE( motorStatus, 6 ) );% not switch on disabled (bit6)
    end
	
%% helper functions
    function bResult = checkIfBit_TRUE(value, bitNumber)
        bResult = ( bitand(value,2^bitNumber) == 2^bitNumber );
    end

    function bResult = checkIfBit_FALSE(value, bitNumber)
        bResult = ( bitand(value,2^bitNumber) == 0 );
    end

end

== stateflow chart MazeGame_full/StateMachine/Chart ==
  state INIT
    resetTwinSafe = false;
    errorAcknowledgeTwinSafe = false;
    motorControl = cmdEl72x1_FAULT_RESET;
    enableApplicationTwinSAFE = false;
    allowVelocityControl = false;
    runTwinSafe=true;
  state TURNING_ON
    state ENABLING_TWINSAFE_POWER_BEFORE_RESET
      motorControl = cmdEl72x1_STOP;
      enableApplicationTwinSAFE = true;
    state RESETTING_TWINSAFE_POWER_SWITCH
      resetTwinSafe = true;
    state ENABLING_TWINSAFE_POWER_AFTER_RESET
      resetTwinSafe = false;
    state PREPARING_SWITCH_ON
      motorControl = cmdEl72x1_VOLTAGE_AND_RELEASE;
    state SWITCHING_ON
      motorControl = cmdEl72x1_SWITCH_ON;
    state ENABLING_OPERATION
      motorControl = cmdEl72x1_ENABLE_OPERATION;
    (default) -> ENABLING_TWINSAFE_POWER_BEFORE_RESET
    ENABLING_TWINSAFE_POWER_BEFORE_RESET -> RESETTING_TWINSAFE_POWER_SWITCH : after(0.4, sec)
    RESETTING_TWINSAFE_POWER_SWITCH -> ENABLING_TWINSAFE_POWER_AFTER_RESET : after(0.1, sec)
    ENABLING_TWINSAFE_POWER_AFTER_RESET -> PREPARING_SWITCH_ON [order 2] : [after(0.1, sec) && stateConditionMotorsSummary.bSwitchOnDisabled]
    PREPARING_SWITCH_ON -> SWITCHING_ON [order 1] : [after(0.1, sec) && stateConditionMotorsSummary.bReadyToSwitchOn]
    SWITCHING_ON -> ENABLING_OPERATION [order 1] : [stateConditionMotorsSummary.bSwitchedOn]
  state ERROR_ACKNOWLEDGE
    state SENDING_TWINSAFE_NOTRUN
      runTwinSafe=false;
    state SENDING_TWINSAFE_ERROR_ACKNOWLEDGE
      errorAcknowledgeTwinSafe = true;
      runTwinSafe=true;
    state RESETTING_MOTOR_DRIVES
      errorAcknowledgeTwinSafe = false;
    (default) -> SENDING_TWINSAFE_NOTRUN
    SENDING_TWINSAFE_NOTRUN -> SENDING_TWINSAFE_ERROR_ACKNOWLEDGE : after(0.1,sec)
    SENDING_TWINSAFE_ERROR_ACKNOWLEDGE -> RESETTING_MOTOR_DRIVES : after(0.1, sec)
  state ERROR
    resetTwinSafe = false;
    motorControl = cmdEl72x1_STOP;
    enableApplicationTwinSAFE = false;
    allowVelocityControl = false;
  state OPERATION
    allowVelocityControl = true;
  (default) -> INIT
  ERROR -> INIT : after(1, sec)
  RESETTING_MOTOR_DRIVES -> INIT : after(0.1, sec)
  INIT -> ERROR_ACKNOWLEDGE [order 2] : [errorTwinSafe || errorSimulink]
  INIT -> INIT [order 1] : [~cmdSwitchOn]
  INIT -> TURNING_ON [order 3] : after(0.1, sec)
  TURNING_ON -> ERROR : [~cmdSwitchOn || errorSimulink]
  ENABLING_TWINSAFE_POWER_AFTER_RESET -> ERROR [order 1] : after(5, sec)
  PREPARING_SWITCH_ON -> ERROR [order 2] : after(5, sec)
  SWITCHING_ON -> ERROR [order 2] : after(5, sec)
  ENABLING_OPERATION -> OPERATION : [stateConditionMotorsSummary.bOperationEnabled]
  OPERATION -> ERROR : [~cmdSwitchOn || errorSimulink ||~twinSafePowerSwitchForDrivesOn]
  data: runTwinSafe output boolean size=1; errorSimulink input boolean; errorTwinSafe input boolean; resetTwinSafe output boolean; errorAcknowledgeTwinSafe output boolean; motorControl output; enableApplicationTwinSAFE output boolean; cmdSwitchOn input boolean; stateConditionMotorsSummary input Bus: StateConditionMotorsSummary; twinSafePowerSwitchForDrivesOn input boolean; cmdEl72x1_STOP parameter double; allowVelocityControl output boolean; cmdEl72x1_ENABLE_OPERATION parameter double; cmdEl72x1_FAULT_RESET parameter double; cmdEl72x1_SWITCH_ON parameter double; cmdEl72x1_VOLTAGE_AND_RELEASE parameter double

== matlab function MazeGame_full/StateMachine/summarizeMotorStateConditions ==
  data: stateConditionMotors input Bus: StateConditionMotors size=1; stateConditionMotorsSummary output Bus: StateConditionMotorsSummary size=1
function stateConditionMotorsSummary = summarizeMotorStateConditions(stateConditionMotors)
%2019-05-28 Nicolas Gerig

%this can be used to ignore some motors by number, in case of
%disconnection.
bIgnoreMotors = false( length(stateConditionMotors), 1 );

%% outputs:
stateConditionMotorsSummary.bSwitchOnDisabled = summarizeStatesWithIgnore(stateConditionMotors.bSwitchOnDisabled, bIgnoreMotors);
stateConditionMotorsSummary.bReadyToSwitchOn = summarizeStatesWithIgnore(stateConditionMotors.bReadyToSwitchOn, bIgnoreMotors);
stateConditionMotorsSummary.bSwitchedOn = summarizeStatesWithIgnore(stateConditionMotors.bSwitchedOn, bIgnoreMotors);
stateConditionMotorsSummary.bOperationEnabled = summarizeStatesWithIgnore(stateConditionMotors.bOperationEnabled, bIgnoreMotors);

%% helper function
    function bSummary = summarizeStatesWithIgnore(states, bIgnoreMotors)
        overWriteTrue = true( length(states) ,1 );
        states(bIgnoreMotors) = overWriteTrue(bIgnoreMotors);
        bSummary = ( sum(states) == length(states) );
    end

end
